simulink model "chap02_113"  (R2020a)
settings: Solver=ode3  StartTime=0.0  StopTime=10.0  RelTol=1e-3
libraries: simulink x1
settings Model: Creator=chen_w3  LastModifiedBy=chen_w3

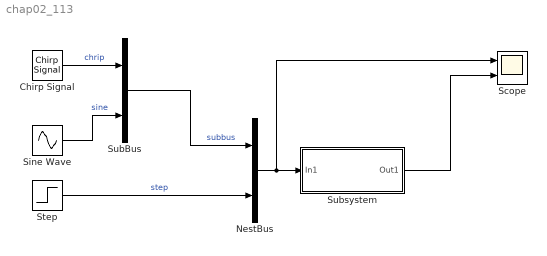
== system chap02_113 ==
  Chirp Signal : simulink/Sources/Chirp Signal  f1=0.1  T=100  f2=1
  NestBus : BusCreator  Inputs=2
  Scope : Scope  NumInputPorts=2
  Sine Wave : Sin  SampleTime=0
  Step : Step  SampleTime=0
  SubBus : BusCreator  Inputs=2
  Subsystem : Subsystem
  wires:
  Step/1 -> NestBus/2  "step"
  Chirp Signal/1 -> SubBus/1  "chrip"
  Sine Wave/1 -> SubBus/2  "sine"
  Subsystem/1(Out1) -> Scope/2
  SubBus/1 -> NestBus/1  "subbus"
  NestBus/1 -> Scope/1, Subsystem/1(In1)

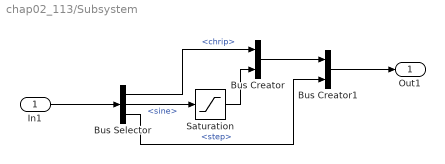
== system chap02_113/Subsystem ==
  In1 : Inport
  Bus Creator : BusCreator  Inputs=2
  Bus Creator1 : BusCreator  Inputs=2
  Bus Selector : BusSelector  OutputSignals=subbus.chrip,subbus.sine,step
  Saturation : Saturate  LowerLimit=-inf
  Out1 : Outport
  wires:
  In1/1 -> Bus Selector/1
  Bus Creator/1 -> Bus Creator1/1
  Bus Creator1/1 -> Out1/1
  Saturation/1 -> Bus Creator/2
  Bus Selector/3 -> Bus Creator1/2  "<step>"
  Bus Selector/1 -> Bus Creator/1  "<chrip>"
  Bus Selector/2 -> Saturation/1  "<sine>"
